simulink library "navlib"  (Simulink 2.09)

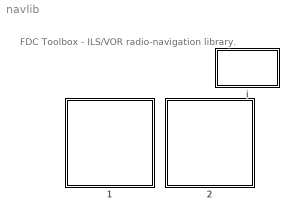
== system navlib ==
  note: FDC Toolbox - ILS/VOR
      | radio-navigation library.
  1 : Subsystem
      settings: OpenFcn=navlib1
      mask Display: disp('ILS signals\nincluding\nsteady-state\nand noise\nerrors')
  2 : Subsystem
      settings: OpenFcn=navlib2
      mask Display: disp('VOR signals\nincluding\nerrors')
  i : Subsystem
      mask Display: disp('???\nMore Info')

== system navlib/1 ==

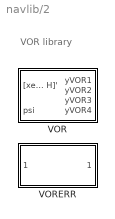
== system navlib/2 ==
  note: VOR library
  VOR : Subsystem  mask(VOR){@1=10000, @2=10000, @3=0, @4=15}
      mask prompts: @1 "x-position VOR at t=0 sec. [m]:"; @2 "y-position VOR at t=0 sec. [m]:"; @3 "Altitude of VOR in [m] above sea level:"; @4 "Course Datum [deg] (0 = north):"
      mask help:
      | Calculation of nominal
      | VOR signals
      mask init:
      | xVOR=@1; yVOR=@2; HVOR=@3; CD=@4*pi/180;
      mask Help: Unmask this block, or type HELP VOR\nat the Matlab command line for more info.
      mask Display: disp('Nominal VOR\nsignals')
  VORERR : Subsystem  mask(VOR error){@1=5}
      mask prompts: @1 "Overall VOR system error [%]:"
      mask help: Steady-state error VOR
      mask init:
      | KVORerr = 1 + (@1/100)
      mask Help: Unmask this block, or type HELP VORERR\nat the Matlab command line for more info.
      mask Display: disp('VOR Steady-\nstate error')

== system navlib/i ==
  note: The basic blocks have been masked. If you don't know
      | the original block-name anymore, press the HELP
      | button. The blocks can be examined more closely if
      | they are 'unmasked'.
  note: On-line help is available from the MATLAB command
      | line: type FDCHELP <blockname> at the command
      | line. For large systems, it is better to abbreviate the
      | block names, to avoid excessive file sizes. See the blocks
      | from the system BEAVER for an example.
  note: This library contains  models for the ILS and VOR
      | systems, including steady-state errors and noise.
  note: Block library of ILS and VOR models

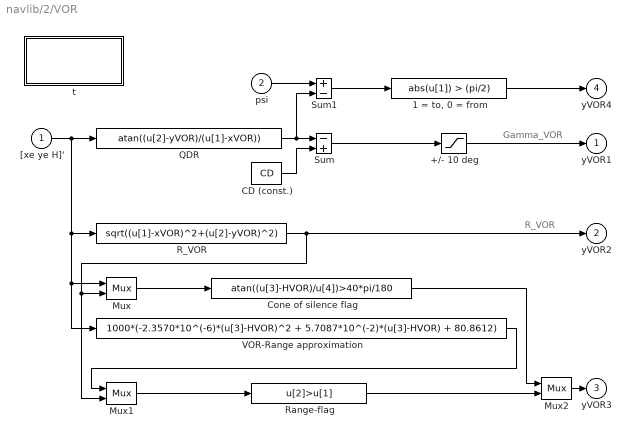
== system navlib/2/VOR ==
  note: R_VOR
  note: Gamma_VOR
  "[xe ye H]'" : Inport  Port=1  PortWidth=-1  SampleTime=-1
  psi : Inport  Port=2  PortWidth=-1  SampleTime=-1
  +/- 10 deg : Saturate  UpperLimit=10*pi/180  LowerLimit=-10*pi/180
  "1 = to, 0 = from" : Fcn  Expr=abs(u[1]) > (pi/2)
  CD (const.) : Constant  Value=CD
  Cone of silence flag : Fcn  Expr=atan((u[3]-HVOR)/u[4])>40*pi/180
  Mux : Mux  Inputs=[3 1]
  Mux1 : Mux  Inputs=2
  Mux2 : Mux  Inputs=2
  QDR : Fcn  Expr=atan((u[2]-yVOR)/(u[1]-xVOR))
  R_VOR : Fcn  Expr=sqrt((u[1]-xVOR)^2+(u[2]-yVOR)^2)
  Range-flag : Fcn  Expr=u[2]>u[1]
  Sum : Sum  Inputs=-+
  Sum1 : Sum  Inputs=+-
  VOR-Range approximation : Fcn  Expr=1000*(-2.3570*10^(-6)*(u[3]-HVOR)^2 + 5.7087*10^(-2)*(u[3]-HVOR) + 80.8612)
  t : Subsystem
      mask Display: disp('VOR signals\nMarc Rauw\nDec 1995')
  yVOR1 : Outport  Port=1  InitialOutput=0
  yVOR2 : Outport  Port=2  InitialOutput=0
  yVOR3 : Outport  Port=3  InitialOutput=0
  yVOR4 : Outport  Port=4  InitialOutput=0
  wires:
  "1 = to, 0 = from"/1 -> yVOR4/1
  CD (const.)/1 -> Sum/2
  Mux/1 -> Cone of silence flag/1
  "[xe ye H]'"/1 -> R_VOR/1, VOR-Range approximation/1, Mux/1, QDR/1
  R_VOR/1 -> Mux1/2, Mux/2, yVOR2/1
  Mux1/1 -> Range-flag/1
  Range-flag/1 -> Mux2/2
  VOR-Range approximation/1 -> Mux1/1
  Mux2/1 -> yVOR3/1
  Cone of silence flag/1 -> Mux2/1
  QDR/1 -> Sum1/2, Sum/1
  psi/1 -> Sum1/1
  Sum1/1 -> "1 = to, 0 = from"/1
  +/- 10 deg/1 -> yVOR1/1
  Sum/1 -> +/- 10 deg/1

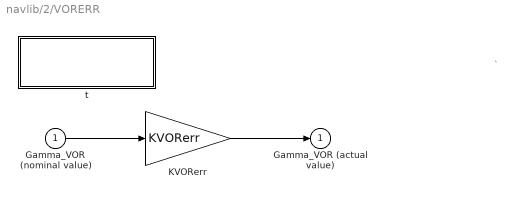
== system navlib/2/VORERR ==
  note: `
  Gamma_VOR (nominal value) : Inport  Port=1  PortWidth=-1  SampleTime=-1
  KVORerr : Gain  Gain=KVORerr
  t : Subsystem
      mask Display: disp('VOR steady-state error\nMarc Rauw\nDec 1995')
  Gamma_VOR (actual value) : Outport  Port=1  InitialOutput=0
  wires:
  KVORerr/1 -> Gamma_VOR (actual value)/1
  Gamma_VOR (nominal value)/1 -> KVORerr/1

== system navlib/2/VOR/t ==
  note: T

== system navlib/2/VORERR/t ==
  note: T
